simulink model "systemSimulation"  (R2025b)
settings: Solver=VariableStepAuto  StartTime=0.0  StopTime=10.0  RelTol=1e-3
libraries: arduinolib x2
settings Model: Creator=erayacikgz  LastModifiedBy=erayacikgz

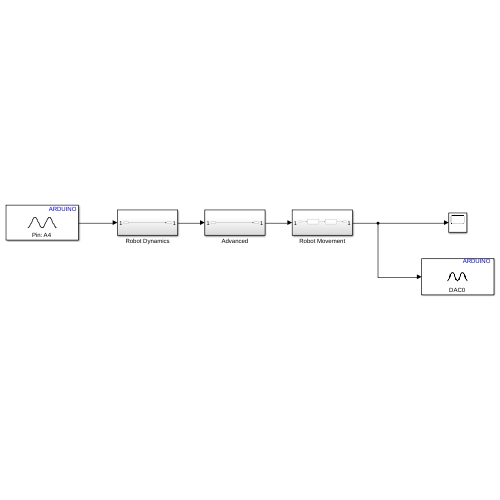
[thumbnail: Simulink's stored preview of the top-level diagram]
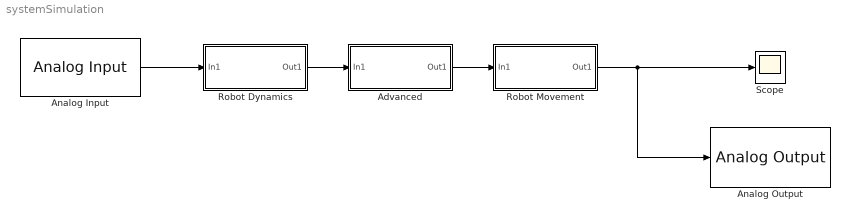
== system systemSimulation ==
  Advanced : Subsystem
  Analog Input : arduinolib/Analog Input  pinNumber=4  ReadResultsOnly=off  ConversionTriggerSource=Software  ExternalTriggerType=uint32( 0 )  OutputDataType=uint16  EnableConversionCompleteNotify=off  EnableOuputStatus=off  SampleTime=-1  blockPlatform=arduino
  Analog Output : arduinolib/Analog Output  blockPlatform=ARDUINO  DACpin=DAC0
  Robot Dynamics : Subsystem
  Robot Movement : Subsystem
  Scope : Scope
  wires:
  Robot Dynamics/1(Out1) -> Advanced/1(In1)
  Robot Movement/1(Out1) -> Analog Output/1, Scope/1
  Analog Input/1 -> Robot Dynamics/1(In1)
  Advanced/1(Out1) -> Robot Movement/1(In1)

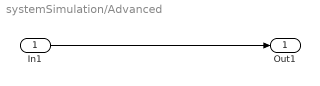
== system systemSimulation/Advanced ==
  In1 : Inport
  Out1 : Outport
  wires:
  In1/1 -> Out1/1

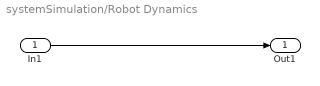
== system systemSimulation/Robot Dynamics ==
  In1 : Inport
  Out1 : Outport
  wires:
  In1/1 -> Out1/1

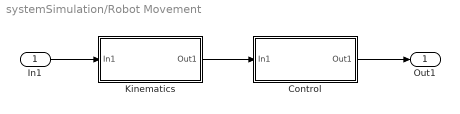
== system systemSimulation/Robot Movement ==
  In1 : Inport
  Control : Subsystem
  Kinematics : Subsystem
  Out1 : Outport
  wires:
  In1/1 -> Kinematics/1(In1)
  Control/1(Out1) -> Out1/1
  Kinematics/1(Out1) -> Control/1(In1)

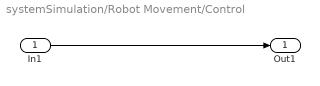
== system systemSimulation/Robot Movement/Control ==
  In1 : Inport
  Out1 : Outport
  wires:
  In1/1 -> Out1/1

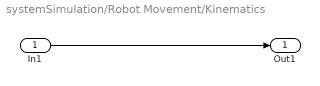
== system systemSimulation/Robot Movement/Kinematics ==
  In1 : Inport
  Out1 : Outport
  wires:
  In1/1 -> Out1/1
